simulink model "ADRC_2RD_plant"  (Simulink 7.1)
settings: Solver=ode45  StartTime=0.0  StopTime=inf  RelTol=1e-3
libraries: ADRC x3, opclib x3, simulink x1
settings Model: Creator=Administrator  LastModifiedBy=Administrator
settings OptimizationCC: InitFltsAndDblsToZero=off
settings DebuggingCC: AlgebraicLoopMsg=none  SolverPrmCheckMsg=none  StrictBusMsg=ErrorLevel1

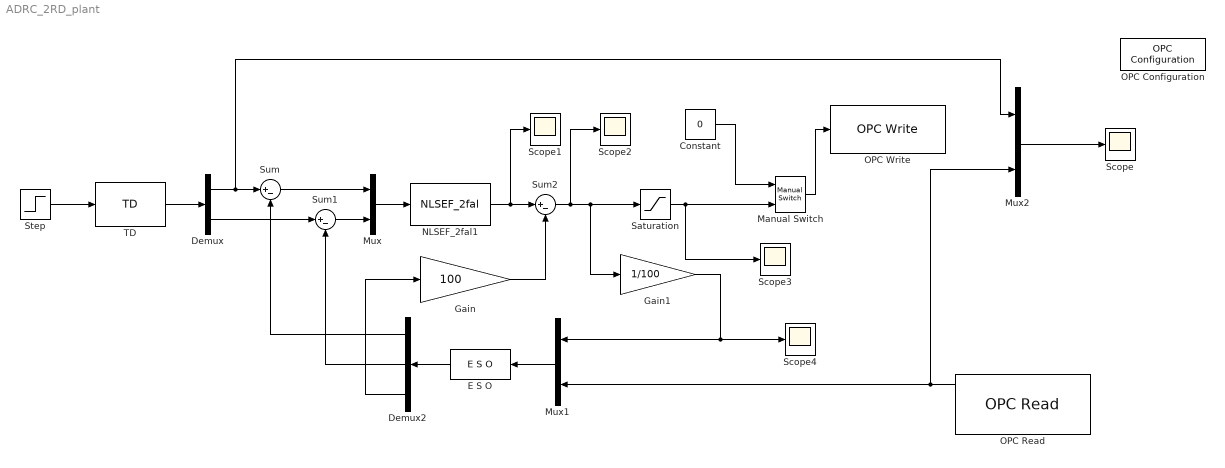
== system ADRC_2RD_plant ==
  Constant : Constant  Value=0  OutDataType=sfix(16)  OutScaling=2^0
  Demux : Demux  Outputs=2
  Demux2 : Demux  Orientation=left  Outputs=3
  E S O : ADRC/ESO/E S O  Orientation=left  Delta=0.1  h=0.1  BB=[20,30,10]
  Gain : Gain  Gain=100
  Gain1 : Gain  Gain=1/100  ParameterDataType=sfix(16)  ParameterScaling=2^0  OutDataType=sfix(16)  OutScaling=2^0
  Manual Switch : simulink/Signal Routing/Manual Switch  SystemSampleTime=-1  sw=1  action=0  varsize=off
  Mux : Mux  Inputs=2
  Mux1 : Mux  Orientation=left  Inputs=2
  Mux2 : Mux  Inputs=2
  NLSEF_2fal1 : ADRC/NLSEF/NLSEF_2fal  Beta1=30  Beta2=25  A1=0.75  A2=1.5  Delta=0.5
  OPC Configuration : opclib/OPC Configuration  opcServers=localhost/OPCServer.WinCC/10  errMissingItems=Error  errReadWrite=Warn  errShutdown=Error  errRTViolation=Warn  rtEnable=on  speedup=1  showLatency=off  beingUsed=on
  OPC Read : opclib/OPC Read  Orientation=left  serverHost=localhost  serverID=OPCServer.WinCC  itemIDs=shuiwei1  readMode=Synchronous (cache)  dataType=double  updateRate=0.1  showQual=on  showTS=on  tsMode=Seconds since start
  OPC Write : opclib/OPC Write  serverHost=localhost  serverID=OPCServer.WinCC  itemIDs=beng2  writeMode=Synchronous  updateRate=0
  Saturation : Saturate  UpperLimit=100  LowerLimit=0  OutDataType=sfix(16)  OutScaling=2^0
  Scope{,1..4} (5 alike) : Scope
      Scope settings: TimeRange=100  YMin=0  YMax=30  SaveName=waterlevel
      Scope1 settings: TimeRange=50  YMin=120  YMax=220
      Scope2 settings: TimeRange=10  YMin=-1300  YMax=200  SaveName=ScopeData2
      Scope3 settings: TimeRange=100  YMin=0  YMax=100  SaveName=ScopeData3
      Scope4 settings: TimeRange=10  YMin=0.25  YMax=3.5  SaveName=ScopeData4
  Step : Step  Time=0  After=12  SampleTime=0
  Sum : Sum  Inputs=|+-
  Sum1 : Sum  Inputs=|+-
  Sum2 : Sum  Inputs=|+-
  TD : ADRC/TD/TD  r0=0.01  h=0.1
  wires:
  Step/1 -> TD/1
  TD/1 -> Demux/1
  Mux/1 -> NLSEF_2fal1/1
  Demux/1 -> Sum/1, Mux2/1
  Demux/2 -> Sum1/1
  E S O/1 -> Demux2/1
  Mux1/1 -> E S O/1
  Demux2/1 -> Sum/2
  Demux2/2 -> Sum1/2
  Sum/1 -> Mux/1
  Sum1/1 -> Mux/2
  NLSEF_2fal1/1 -> Sum2/1, Scope1/1
  Demux2/3 -> Gain/1
  Gain/1 -> Sum2/2
  Sum2/1 -> Scope2/1, Gain1/1, Saturation/1
  Mux2/1 -> Scope/1
  Gain1/1 -> Mux1/1, Scope4/1
  OPC Read/1 -> Mux1/2, Mux2/2
  Manual Switch/1 -> OPC Write/1
  Constant/1 -> Manual Switch/1
  Saturation/1 -> Manual Switch/2, Scope3/1
